simulink model "gpt_rdf2"  (R2013b)
settings: Solver=FixedStepDiscrete  StartTime=0.0  StopTime=4  FixedStep=1/800  RelTol=1e-3
libraries: commanapbnd3 x5
settings Model: Creator=rmg37  LastModifiedBy=rmg37
settings DataIOCC: SaveOutput=off  SaveTime=off
settings OptimizationCC: LocalBlockOutputs=off
settings DebuggingCC: AlgebraicLoopMsg=error  SingleTaskRateTransMsg=error

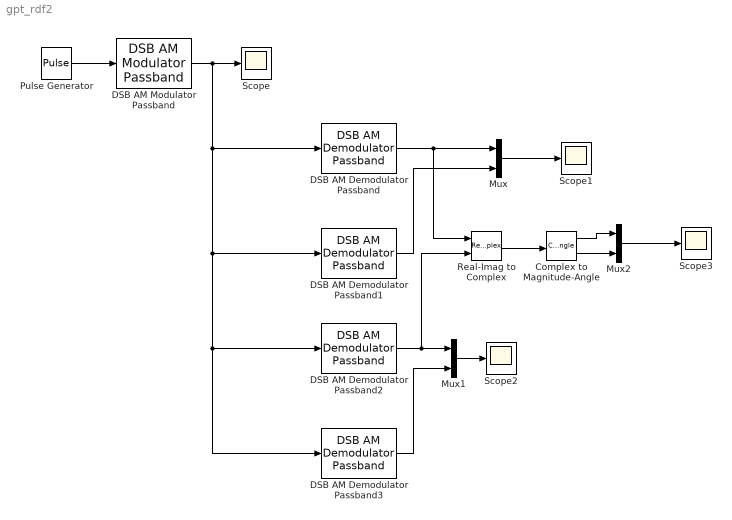
== system gpt_rdf2 ==
  Complex to Magnitude-Angle : ComplexToMagnitudeAngle
  DSB AM Demodulator Passband : commanapbnd3/DSB AM Demodulator Passband  Fc=100  Ph=0  method=Butterworth  n=4  cf=4  Rp=0.1  Rs=50  Offset=0
  DSB AM Demodulator Passband1 : commanapbnd3/DSB AM Demodulator Passband  Fc=100  Ph=pi/2  method=Butterworth  n=4  cf=4  Rp=0.1  Rs=50  Offset=0
  DSB AM Demodulator Passband2 : commanapbnd3/DSB AM Demodulator Passband  Fc=100  Ph=pi/4  method=Butterworth  n=4  cf=4  Rp=0.1  Rs=50  Offset=0
  DSB AM Demodulator Passband3 : commanapbnd3/DSB AM Demodulator Passband  Fc=100  Ph=3*pi/4  method=Butterworth  n=4  cf=4  Rp=0.1  Rs=50  Offset=0
  DSB AM Modulator Passband : commanapbnd3/DSB AM Modulator Passband  Fc=100  Ph=0  Offset=0
  Mux : Mux  Inputs=2
  Mux1 : Mux  Inputs=2
  Mux2 : Mux  Inputs=2
  Pulse Generator : DiscretePulseGenerator  PulseType=Time based  PulseWidth=50
  Real-Imag to Complex : RealImagToComplex
  Scope{,1..3} (4 alike) : Scope
      Scope2 settings: SaveName=ScopeData2
      Scope3 settings: SaveName=ScopeData3
  wires:
  Pulse Generator/1 -> DSB AM Modulator Passband/1
  DSB AM Demodulator Passband/1 -> Real-Imag to Complex/1, Mux/1
  Mux/1 -> Scope1/1
  DSB AM Demodulator Passband1/1 -> Mux/2
  DSB AM Modulator Passband/1 -> DSB AM Demodulator Passband3/1, DSB AM Demodulator Passband2/1, DSB AM Demodulator Passband1/1, DSB AM Demodulator Passband/1, Scope/1
  DSB AM Demodulator Passband2/1 -> Real-Imag to Complex/2, Mux1/1
  Mux1/1 -> Scope2/1
  DSB AM Demodulator Passband3/1 -> Mux1/2
  Real-Imag to Complex/1 -> Complex to Magnitude-Angle/1
  Mux2/1 -> Scope3/1
  Complex to Magnitude-Angle/2 -> Mux2/2
  Complex to Magnitude-Angle/1 -> Mux2/1
